simulink model "oscillator_roessler"  (R2023b)
settings: Solver=VariableStepAuto  StartTime=0.0  StopTime=100  RelTol=1e-3
settings Model: Creator=awcm9  LastModifiedBy=awcm9

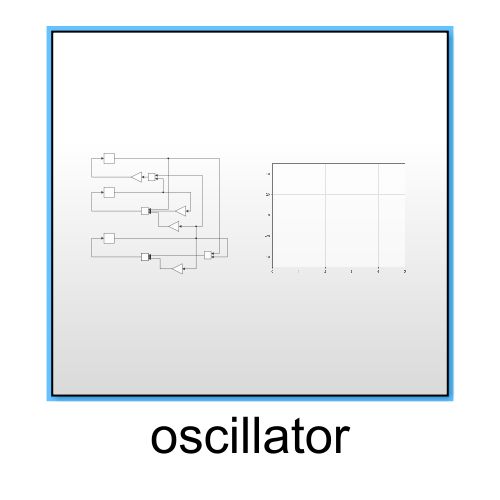
[thumbnail: Simulink's stored preview of the top-level diagram]
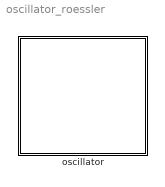
== system oscillator_roessler ==
  oscillator : Subsystem

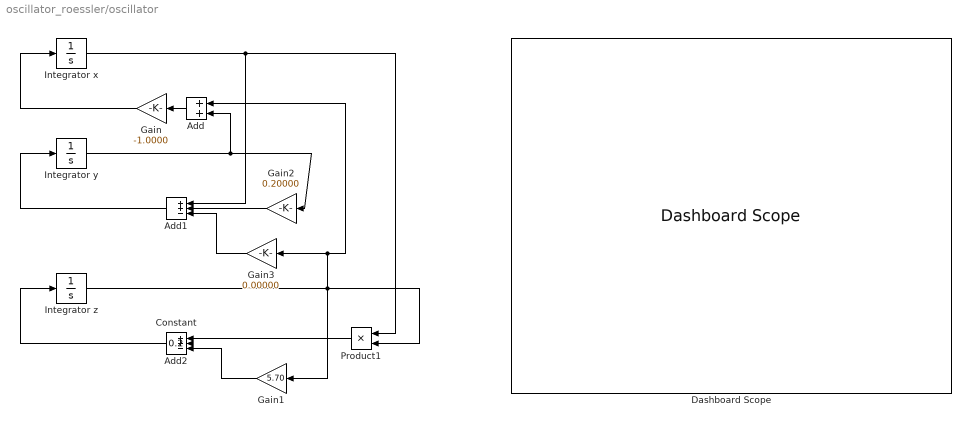
== system oscillator_roessler/oscillator ==
  Add : Sum
  Add1 : Sum  Inputs=++-
  Add2 : Sum  Inputs=++-
  Constant : Constant  Value=0.2
  Dashboard Scope : DashboardScope  ShowInitialText=off  TimeSpan=5  Ymin=-50  Ymax=50  ScaleAtStop=off
  Gain : Gain  Gain=-1.0000
  Gain1 : Gain  Gain=5.70
  Gain2 : Gain  Gain=0.20000
  Gain3 : Gain  Gain=0.00000
  Integrator x : Integrator  InitialCondition=1
  Integrator y : Integrator
  Integrator z : Integrator
  Product1 : Product
  wires:
  Constant/1 -> Add2/2
  Gain1/1 -> Add2/3
  Add2/1 -> Integrator z/1
  Product1/1 -> Add2/1
  Add1/1 -> Integrator y/1
  Gain3/1 -> Add1/3
  Gain2/1 -> Add1/2
  Gain/1 -> Integrator x/1
  Integrator z/1 -> Add/1, Gain3/1, Gain1/1, Product1/2
  Add/1 -> Gain/1
  Integrator x/1 -> Product1/1, Add1/1
  Integrator y/1 -> Add/2, Gain2/1
